simulink model "Simulation_GSM_out_2015a"  (R2015a)
settings: Solver=ode15s  StartTime=0.0  StopTime=14  MaxStep=1e-3  RelTol=1e-5  AbsTol=1e-4
Description:
  | Testdatei zur Verifikation des Modells GSM mit Propeller
settings Model: CovSFcnEnable=off  Creator=wke  LastModifiedBy=sg
settings DataIOCC: SignalLoggingSaveFormat=ModelDataLogs
settings OptimizationCC: ExpressionDepthLimit=2147483647  InitFltsAndDblsToZero=on
settings DebuggingCC: SaveWithParameterizedLinksMsg=none  UnderspecifiedInitializationDetection=Classic  MergeDetectMultiDrivingBlocksExec=none  SolverPrmCheckMsg=warning  FcnCallInpInsideContextMsg=EnableAllAsWarning  StateNameClashWarn=warning
settings GRTTargetCC: CombineOutputUpdateFcns=off  GRTInterface=on

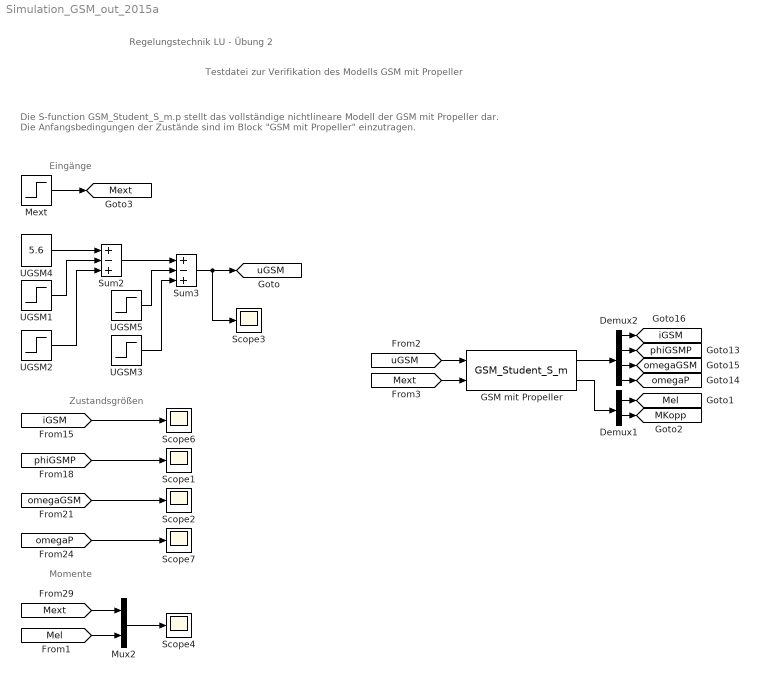
== system Simulation_GSM_out_2015a ==
  note: Eingänge
  note: Zustandsgrößen
  note: Momente
  note: Testdatei zur Verifikation des Modells GSM mit Propeller
  note: Die S-function GSM_Student_S_m.p stellt das vollständige nichtlineare Modell
      | der GSM mit Propeller dar. Die Anfangsbedingungen der Zustände sind im Block
      | "GSM mit Propeller" einzutragen.
  note: Regelungstechnik LU - Übung 2
  Demux1 : Demux  Outputs=2
  Demux2 : Demux
  GSM mit Propeller : M-S-Function  FunctionName=GSM_Student_S_m  Parameters=iGSM_0,phiGSMP_0,omegaGSM_0,omegaP_0  mask{iGSM_0=0, phiGSMP_0=0, omegaGSM_0=0, omegaP_0=0}
      mask prompts: iGSM_0 "Anfangsbedingung iGSM"; phiGSMP_0 "Anfangsbedingung phiGSMP"; omegaGSM_0 "Anfangsbedingung omegaGSM"; omegaP_0 "Anfangsbedingung omegaP"
  Mext : Step  Time=11  After=0.25  SampleTime=0
  Mux2 : Mux  Inputs=2
  Scope{1..4,6..7} (6 alike) : Scope
      Scope1 settings: TimeRange=auto  MaxDataPoints=5000  SaveToWorkspace=off  SaveName=ScopeData  YMin=-0.25  YMax=0.85  SampleTime=-1
      Scope2 settings: TimeRange=14  MaxDataPoints=5000  SaveToWorkspace=off  YMin=0  YMax=1700  SampleTime=-1
      Scope3 settings: TimeRange=auto  MaxDataPoints=5000  SaveToWorkspace=off  SaveName=ScopeData3  YMin=3.5  YMax=5.6  SampleTime=-1
      Scope4 settings: TimeRange=auto  MaxDataPoints=5000  SaveToWorkspace=off  SaveName=ScopeData4  YMin=0  YMax=1.4  SampleTime=-1
      Scope6 settings: TimeRange=auto  MaxDataPoints=5000  SaveToWorkspace=off  SaveName=ScopeData5  YMin=-3  YMax=8.5  SampleTime=-1
      Scope7 settings: TimeRange=14  MaxDataPoints=5000  SaveToWorkspace=off  SaveName=ScopeData2  YMin=0  YMax=30  SampleTime=-1
  Sum2 : Sum  Inputs=+-+
  Sum3 : Sum  Inputs=+-+
  UGSM1 : Step  Time=2  SampleTime=0
  UGSM2 : Step  Time=5  SampleTime=0
  UGSM3 : Step  Time=13  After=2  SampleTime=0
  UGSM4 : Constant  Value=5.6
  UGSM5 : Step  Time=8  After=2  SampleTime=0
  tag scope: MKopp=global, Mel=global, Mext=global, iGSM=global, omegaGSM=global, omegaP=global, phiGSMP=global, uGSM=global
  wires:
  [uGSM] -> GSM mit Propeller/1
  [Mext] -> GSM mit Propeller/2
  Demux2/1 -> [iGSM]
  Demux2/2 -> [phiGSMP]
  Demux2/3 -> [omegaGSM]
  Demux2/4 -> [omegaP]
  GSM mit Propeller/1 -> Demux2/1
  GSM mit Propeller/2 -> Demux1/1
  Demux1/1 -> [Mel]
  Demux1/2 -> [MKopp]
  Mext/1 -> [Mext]
  UGSM4/1 -> Sum2/1
  UGSM1/1 -> Sum2/2
  Sum2/1 -> Sum3/1
  Sum3/1 -> [uGSM], Scope3/1
  UGSM2/1 -> Sum2/3
  UGSM5/1 -> Sum3/2
  UGSM3/1 -> Sum3/3
  Mux2/1 -> Scope4/1
  [iGSM] -> Scope6/1
  [phiGSMP] -> Scope1/1
  [omegaGSM] -> Scope2/1
  [omegaP] -> Scope7/1
  [Mext] -> Mux2/1
  [Mel] -> Mux2/2
